simulink model "Proj_16_10"  (R2020a)
settings: Solver=VariableStepAuto  StartTime=0.0  StopTime=10.0  RelTol=1e-3
undefined symbols (not defined in the file): T
settings Model: Creator=jguil  LastModifiedBy=jguil

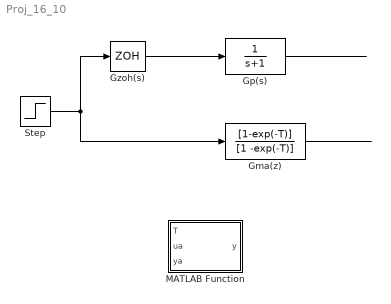
== system Proj_16_10 ==
  Gma(z) : DiscreteTransferFcn  Numerator=[1-exp(-T)]  Denominator=[1 -exp(-T)]
  Gp(s) : TransferFcn  Denominator=[1 1]
  Gzoh(s) : ZeroOrderHold  SampleTime=-1
  MATLAB Function : MATLAB Function  TreatAsAtomicUnit=on
  Step : Step  SampleTime=0
  wires:
  Gzoh(s)/1 -> Gp(s)/1
  Step/1 -> Gma(z)/1, Gzoh(s)/1
  Gma(z)/1 -> ?
  Gp(s)/1 -> ?

== matlab function Proj_16_10/MATLAB Function ==
  data: T input; y output; ua input; ya input
function y = ModeloSW(T,ua,ya)

a = 1-exp(-T);
b=exp(-T);

y = a*ua+b*ya;
